simulink model "openLoop2PIBC"  (R2021a)
settings: Solver=ode23t  StartTime=0.0  StopTime=0.5  RelTol=1e-3
undefined symbols (not defined in the file or in its folder): plecs
settings Model: Creator=qaromose  LastModifiedBy=qaromose

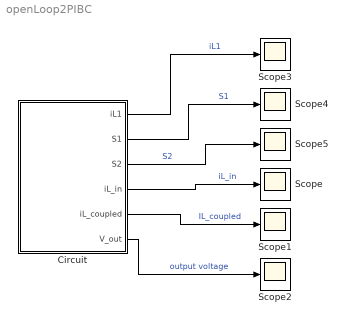
== system openLoop2PIBC ==
  Circuit : Subsystem  LoadFcn=plecs('sl', 200);  InitFcn=plecs('sl', 214);  StartFcn=plecs('sl', 208);  StopFcn=plecs('sl', 209);  mask(PlecsCircuit){PLECSData=<binary blob, 4060 chars, not shown>}
      mask prompts: PLECSData "PLECS Data (Do not delete or modify!)"
      mask init:
      | % PLACE CUSTOM INITIALIZATIONS ABOVE
      | % DO NOT REMOVE
      | plecs('sl', 215);
      | % DO NOT REMOVE
      settings: CopyFcn=plecs('sl', 203);  DeleteFcn=plecs('sl', 205);  UndoDeleteFcn=plecs('sl', 206);  PreSaveFcn=plecs('sl', 211);  PostSaveFcn=plecs('sl', 201);  NameChangeFcn=plecs('sl', 210);  DestroyFcn=plecs('sl', 207);  PreCopyFcn=plecs('sl', 216);  OpenFcn=plecs('sl', 202);  ErrorFcn=plerrorfcn
      mask Help: eval('plecs(''help'', ''qthelp:///creatingacircuit.html'')')
      mask Display: disp('PLECS\nCircuit')
  Scope{,1..5} (6 alike) : Scope
  wires:
  Circuit/3(S2) -> Scope5/1  "S2"
  Circuit/2(S1) -> Scope4/1  "S1"
  Circuit/1(iL1) -> Scope3/1  "iL1"
  Circuit/4(iL_in) -> Scope/1  "iL_in"
  Circuit/5(iL_coupled) -> Scope1/1  "IL_coupled"
  Circuit/6(V_out) -> Scope2/1  "output voltage"

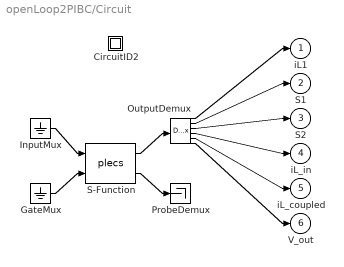
== system openLoop2PIBC/Circuit ==
  " CircuitID2 " : Subsystem
  " GateMux " : Ground
  " InputMux " : Ground
  " OutputDemux " : Demux  Outputs=[ 1 1 1 1 2 1 ]
  " ProbeDemux " : Terminator
  " S-Function " : S-Function  FunctionName=plecs  SFunctionDeploymentMode=off  EnableBusSupport=off
  iL1 : Outport  PortDimensions=1
  S1 : Outport  Port=2  PortDimensions=1
  S2 : Outport  Port=3  PortDimensions=1
  iL_in : Outport  Port=4  PortDimensions=1
  iL_coupled : Outport  Port=5  PortDimensions=2
  V_out : Outport  Port=6  PortDimensions=1
  wires:
  " InputMux "/1 -> " S-Function "/1
  " GateMux "/1 -> " S-Function "/2
  " S-Function "/1 -> " OutputDemux "/1
  " S-Function "/2 -> " ProbeDemux "/1
  " OutputDemux "/1 -> iL1/1
  " OutputDemux "/2 -> S1/1
  " OutputDemux "/3 -> S2/1
  " OutputDemux "/4 -> iL_in/1
  " OutputDemux "/5 -> iL_coupled/1
  " OutputDemux "/6 -> V_out/1

== system openLoop2PIBC/Circuit/ CircuitID2  ==
